simulink model "therapy_BW"  (Simulink 6.6)
settings: Solver=ode45  SolverMode=SingleTasking  StartTime=0.0  StopTime=999999  MaxStep=10  RelTol=1e-3  AbsTol=1e-3
settings Model: Creator=lfd  LastModifiedBy=lfd  ExtModeAutoUpdateStatusClock=off
settings DataIOCC: LimitDataPoints=off  SaveOutput=off  SaveTime=off
settings OptimizationCC: BlockReduction=off  BooleanDataType=off
settings DebuggingCC: SignalResolutionControl=TryResolveAllWithWarning  SolverPrmCheckMsg=none  MultiTaskDSMMsg=warning  MultiTaskCondExecSysMsg=none  StrictBusMsg=None
settings HardwareCC: TargetUnknown=on
settings RTWCC: IncludeERTFirstTime=on
settings STFCustomTargetCC: TargetFcnLib=ansi_tfl_tmw.mat  GenFloatMathFcnCalls=ANSI_C  ModelReferenceCompliant=off  SystemTargetFile=grt.tlc

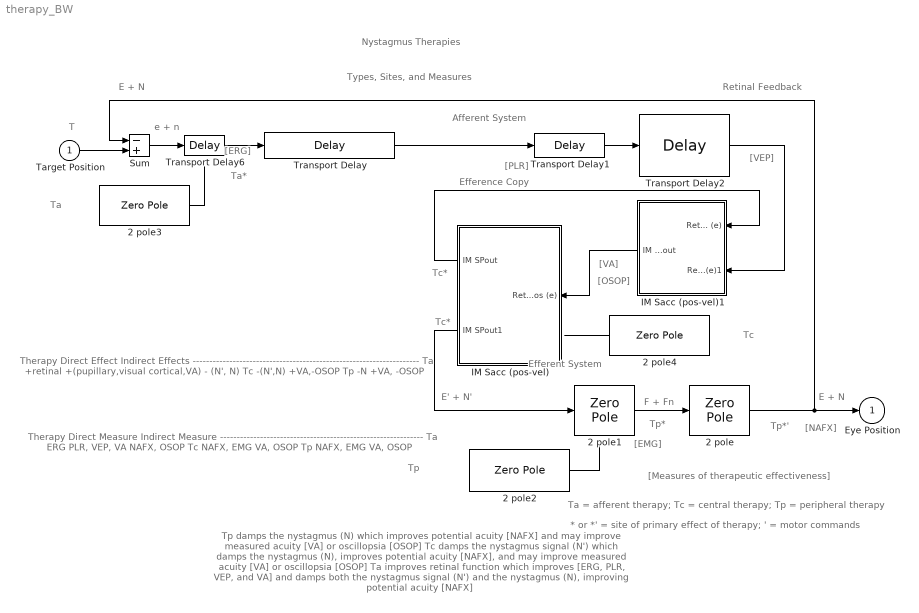
== system therapy_BW ==
  note: Nystagmus Therapies
  note: Retinal Feedback
  note: E + N
  note: e + n
  note: E + N
  note: T
  note: E' + N'
  note: F + Fn
  note: [VA]
  note: Tc
  note: Tp
  note: Ta
  note: Tc*
  note: Ta*
  note: Tp*
  note: Tp*'
  note: [ERG]
  note: [VEP]
  note: [PLR]
  note: Ta = afferent therapy; Tc = central therapy; Tp = peripheral therapy
  note: * or *' = site of primary effect of therapy; ' = motor commands
  note: Tp damps the nystagmus (N) which improves potential acuity [NAFX] and may improve measured acuity [VA] or oscillopsia [OSOP]
      | Tc damps the  nystagmus signal (N') which damps the nystagmus (N), improves potential acuity [NAFX], and may improve measured acuity [VA] or oscillopsia [OSOP]
      | Ta improves retinal function which improves [ERG, PLR, VEP, and VA] and damps both the nystagmus signal (N') and the nystagmus (N), improving potential acuity [NAFX]
  note: [OSOP]
  note: Efference Copy
  note: Tc*
  note: [NAFX]
  note: [Measures of therapeutic effectiveness]
  note: Therapy	            Direct Measure          Indirect Measure
      | -------------------------------------------------------------
      |   Ta                         ERG                                PLR, VEP, VA
      |                                                                 NAFX, OSOP
      | Tc                          NAFX, EMG                  VA, OSOP
      | Tp                         NAFX, EMG                  VA, OSOP
  note: Therapy	                    Direct Effect       Indirect Effects
      | --------------------------------------------------------------------
      | Ta                               +retinal               +(pupillary,visual cortical,VA)
      |                                            - (N', N)
      |         Tc                              -(N',N)                   +VA,-OSOP
      |          Tp                               -N                        +VA, -OSOP
  note: Efferent System
  note: Afferent System
  note: [EMG]
  note: Types, Sites, and Measures
  Target Position : Inport
  2 pole{,1..3} (4 alike) : ZeroPole  Zeros=[ ]  Poles=[ -1/.18 -1/.007]  Gain=[1/.18 * 1/.007]
      2 pole mask Display: disp('Eye')
      2 pole1 mask Display: disp('EOM')
      2 pole2 mask Display: disp('Surgical, Optical\n& Drug Therapies')
      2 pole3 mask Display: disp('Gene\nTherapies')
  2 pole4 : ZeroPole  Orientation=left  Zeros=[ ]  Poles=[ -1/.18 -1/.007]  Gain=[1/.18 * 1/.007]
      mask Display: disp('Neurosurgical\n& Drug Therapies')
  IM Sacc (pos-vel) : Subsystem  Orientation=left
      mask Display: disp('Ocular\nMotor\nSystem')
  IM Sacc (pos-vel)1 : Subsystem  Orientation=left
      mask Display: disp('Higher\nCortical\nCenters')
  Sum : Sum  Inputs=-+  SaturateOnIntegerOverflow=on  InputSameDT=on
  Transport Delay : TransportDelay  DelayTime=0.015
      mask Display: disp('Optic Nerve, Chiasm, Tract')
  Transport Delay1 : TransportDelay  DelayTime=0.015
      mask Display: disp('LGN')
  Transport Delay2 : TransportDelay  DelayTime=0.015
      mask Display: disp('Visual Cortex')
  Transport Delay6 : TransportDelay  DelayTime=0
      mask Display: disp('Retina')
  Eye Position : Outport  InitialOutput=0
  wires:
  2 pole1/1 -> 2 pole/1
  2 pole2/1 -> ?
  2 pole4/1 -> ?
  Target Position/1 -> Sum/2
  Sum/1 -> Transport Delay6/1
  Transport Delay6/1 -> Transport Delay/1
  Transport Delay/1 -> Transport Delay1/1
  Transport Delay1/1 -> Transport Delay2/1
  2 pole/1 -> Eye Position/1, Sum/1
  Transport Delay2/1 -> IM Sacc (pos-vel)1/2(RetErr Pos (e)1)
  IM Sacc (pos-vel)1/1(IM SPout) -> IM Sacc (pos-vel)/1(RetErr Pos (e))
  IM Sacc (pos-vel)/2(IM SPout1) -> 2 pole1/1
  IM Sacc (pos-vel)/1(IM SPout) -> IM Sacc (pos-vel)1/1(RetErr Pos (e))
  ? -> 2 pole4/1
  ? -> 2 pole2/1
  2 pole3/1 -> ?
  ? -> 2 pole3/1

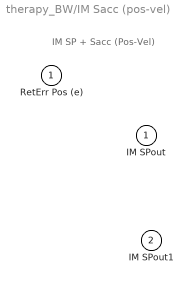
== system therapy_BW/IM Sacc (pos-vel) ==
  note: IM SP + Sacc (Pos-Vel)
  RetErr Pos (e) : Inport
  IM SPout : Outport  InitialOutput=0
  IM SPout1 : Outport  Port=2  InitialOutput=0

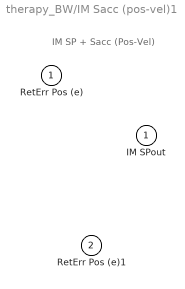
== system therapy_BW/IM Sacc (pos-vel)1 ==
  note: IM SP + Sacc (Pos-Vel)
  RetErr Pos (e) : Inport
  RetErr Pos (e)1 : Inport  Port=2
  IM SPout : Outport  InitialOutput=0
